simulink model "ex3p22"  (R2020a)
settings: Solver=FixedStepAuto  StartTime=0.0  StopTime=inf  FixedStep=0.001  RelTol=1e-3
settings Model: Creator=corte  LastModifiedBy=corte
settings OptimizationCC: EnhancedBackFolding=on  PassReuseOutputArgsAs=Individual arguments  ZeroExternalMemoryAtStartup=off  ZeroInternalMemoryAtStartup=off  MaxStackSize=64  OptimizeBlockOrder=speed  DifferentSizesBufferReuse=on  OptimizationCustomize=off  EfficientTunableParamExpr=on
settings DebuggingCC: ParameterTunabilityLossMsg=error
settings HardwareCC: ProdBitPerPointer=32  ProdBitPerSizeT=32  ProdBitPerPtrDiffT=32  ProdLargestAtomicInteger=Long  ProdLargestAtomicFloat=Double  ProdWordSize=32  ProdHWDeviceType=ARM Compatible->ARM Cortex
settings SFSimCC: MATLABDynamicMemAlloc=off
settings RTWCC: SystemTargetFile=ert.tlc  HardwareBoard=Android Device  TemplateMakefile=ert_default_tmf  RTWVerbose=off  Toolchain=Android SDK/NDK Tools
settings CodeAppCC: ForceParamTrailComments=on  IgnoreCustomStorageClasses=off  OperatorAnnotations=on  SimulinkDataObjDesc=on  SFDataObjDesc=on  InsertBlockDesc=on
settings ERTTargetCC: SupportContinuousTime=on

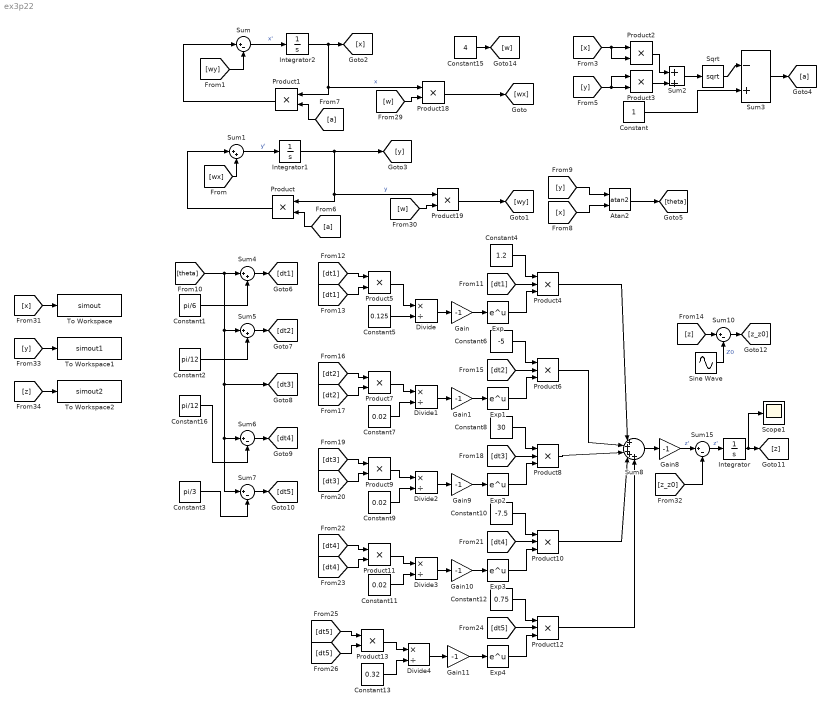
== system ex3p22 ==
  Atan2 : Trigonometry  Operator=atan2
  Constant : Constant
  Constant1 : Constant  Value=pi/6
  Constant10 : Constant  Value=-7.5
  Constant11 : Constant  Value=0.02
  Constant12 : Constant  Value=0.75
  Constant13 : Constant  Value=0.32
  Constant15 : Constant  Value=4
  Constant16 : Constant  Value=pi/12
  Constant2 : Constant  Value=pi/12
  Constant3 : Constant  Value=pi/3
  Constant4 : Constant  Value=1.2
  Constant5 : Constant  Value=0.125
  Constant6 : Constant  Value=-5
  Constant7 : Constant  Value=0.02
  Constant8 : Constant  Value=30
  Constant9 : Constant  Value=0.02
  Divide{,1..4} (5 alike) : Product  Inputs=*/
  Exp{,1..4} (5 alike) : Math  SaturateOnIntegerOverflow=on
  Gain{,1,8..11} (6 alike) : Gain  Gain=-1
  Integrator : Integrator
  Integrator1 : Integrator
  Integrator2 : Integrator  InitialCondition=2
  Product{,1..3,5,7,9,11,13,18..19} (11 alike) : Product
  Product{4,6,8,10,12} (5 alike) : Product  Inputs=3
  Scope1 : Scope
  Sine Wave : Sin  Amplitude=0.15e-3  Frequency=pi/2  SampleTime=0
  Sqrt : Sqrt  SaturateOnIntegerOverflow=on
  Sum{,6..7,10,15} (5 alike) : Sum  Inputs=|+-
  Sum{1..2,4..5} (4 alike) : Sum  Inputs=|++
  Sum3 : Sum  Inputs=|-+
  Sum8 : Sum  Inputs=|+++++
  To Workspace : ToWorkspace  VariableName=simout  SaveFormat=Timeseries  SampleTime=-1
  To Workspace1 : ToWorkspace  VariableName=simout1  SaveFormat=Timeseries  SampleTime=-1
  To Workspace2 : ToWorkspace  VariableName=simout2  SaveFormat=Timeseries  SampleTime=-1
  wires:
  Integrator2/1 -> [x], Product1/1, Product18/1  "x"
  Sum/1 -> Integrator2/1  "x'"
  Constant6/1 -> Product6/1
  Product4/1 -> Sum8/1
  [z] -> To Workspace2/1
  [z_z0] -> Sum15/2
  [dt3] -> Product8/2
  Product11/1 -> Divide3/1
  [wy] -> Sum/2
  Gain8/1 -> Sum15/1  "z'"
  Integrator/1 -> Scope1/1, [z]
  Gain11/1 -> Exp4/1
  Sine Wave/1 -> Sum10/2  "Z0"
  Product5/1 -> Divide/1
  [x] -> To Workspace/1
  Sum6/1 -> [dt4]
  Constant16/1 -> Sum6/2
  Constant15/1 -> [w]
  Exp1/1 -> Product6/3
  Sum10/1 -> [z_z0]
  [a] -> Product/2
  Product8/1 -> Sum8/3
  Product13/1 -> Divide4/1
  Sqrt/1 -> Sum3/1
  Gain9/1 -> Exp2/1
  Sum7/1 -> [dt5]
  Product19/1 -> [wy]
  [w] -> Product18/2
  Exp3/1 -> Product10/3
  [theta] -> Sum7/1, Sum6/1, [dt3], Sum5/1, Sum4/1
  [y] -> To Workspace1/1
  Atan2/1 -> [theta]
  Constant7/1 -> Divide1/2
  [dt3] -> Product9/1
  [w] -> Product19/2
  Product9/1 -> Divide2/1
  [dt4] -> Product10/2
  Sum5/1 -> [dt2]
  Constant13/1 -> Divide4/2
  Sum15/1 -> Integrator/1  "z'"
  Divide3/1 -> Gain10/1
  [dt5] -> Product13/1
  Product6/1 -> Sum8/2
  Product12/1 -> Sum8/5
  Product10/1 -> Sum8/4
  [x] -> Product2/2, Product2/1
  Gain/1 -> Exp/1
  Sum1/1 -> Integrator1/1  "y'"
  [dt5] -> Product13/2
  Constant10/1 -> Product10/1
  Gain1/1 -> Exp1/1
  [dt3] -> Product9/2
  Constant11/1 -> Divide3/2
  [dt4] -> Product11/1
  Divide4/1 -> Gain11/1
  Divide2/1 -> Gain9/1
  Integrator1/1 -> [y], Product19/1, Product/1  "y"
  Constant9/1 -> Divide2/2
  [dt5] -> Product12/2
  [dt4] -> Product11/2
  Divide/1 -> Gain/1
  Constant8/1 -> Product8/1
  [dt1] -> Product5/1
  Product7/1 -> Divide1/1
  [z] -> Sum10/1
  Constant5/1 -> Divide/2
  [dt1] -> Product5/2
  Gain10/1 -> Exp3/1
  [dt2] -> Product6/2
  [a] -> Product1/2
  Exp2/1 -> Product8/3
  [dt2] -> Product7/1
  [dt1] -> Product4/2
  Constant12/1 -> Product12/1
  Divide1/1 -> Gain1/1
  Exp/1 -> Product4/3
  Product18/1 -> [wx]
  [wx] -> Sum1/2
  Constant1/1 -> Sum4/2
  Exp4/1 -> Product12/3
  Sum2/1 -> Sqrt/1
  Constant3/1 -> Sum7/2
  Product3/1 -> Sum2/2
  Constant4/1 -> Product4/1
  Constant/1 -> Sum3/2
  Product1/1 -> Sum/1
  [dt2] -> Product7/2
  Product2/1 -> Sum2/1
  Product/1 -> Sum1/1
  Sum8/1 -> Gain8/1
  [y] -> Atan2/1
  [x] -> Atan2/2
  Sum3/1 -> [a]
  [y] -> Product3/1, Product3/2
  Constant2/1 -> Sum5/2
  Sum4/1 -> [dt1]
